simulink model "MotorPositionControl"  (R2020b)
settings: Solver=ode15s  StartTime=0.0  StopTime=0.2  RelTol=1e-3
undefined symbols (not defined in the file): b, J, kd, ke, ki, kp, kt, L, R
settings Model: DataDictionary=data_dict.sldd  Creator=Shree  LastModifiedBy=Shree

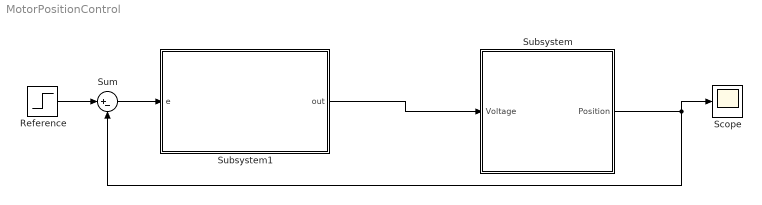
== system MotorPositionControl ==
  "Reference " : Step  Time=0.001  SampleTime=0
  Scope : Scope
  Subsystem : Subsystem
  Subsystem1 : Subsystem
  Sum : Sum  Inputs=|+-
  wires:
  Subsystem/1(Position) -> Scope/1, Sum/2
  Subsystem1/1(out) -> Subsystem/1(Voltage)
  "Reference "/1 -> Sum/1
  Sum/1 -> Subsystem1/1(e)

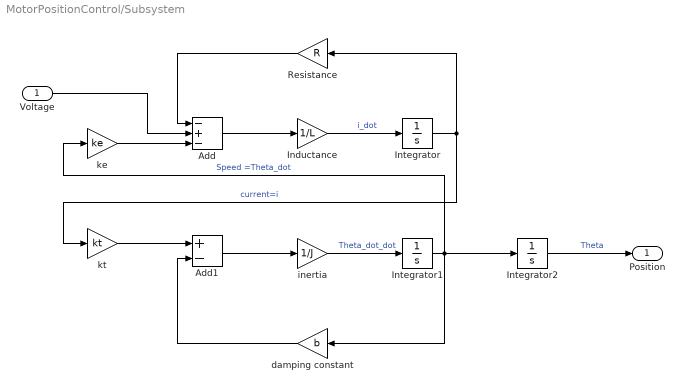
== system MotorPositionControl/Subsystem ==
  Voltage : Inport
  Add : Sum  Inputs=-+-
  Add1 : Sum  Inputs=+-
  Inductance : Gain  Gain=1/L
  Integrator : Integrator
  Integrator1 : Integrator
  Integrator2 : Integrator
  Resistance : Gain  Gain=R
  damping constant : Gain  Gain=b
  inertia : Gain  Gain=1/J
  ke : Gain  Gain=ke
  kt : Gain  Gain=kt
  Position : Outport
  wires:
  Inductance/1 -> Integrator/1  "i_dot"
  inertia/1 -> Integrator1/1  "Theta_dot_dot"
  Add1/1 -> inertia/1
  Integrator1/1 -> Integrator2/1, ke/1, damping constant/1  "Speed =Theta_dot"
  Integrator/1 -> Resistance/1, kt/1  "current=i"
  Resistance/1 -> Add/1
  kt/1 -> Add1/1
  damping constant/1 -> Add1/2
  Add/1 -> Inductance/1
  Integrator2/1 -> Position/1  "Theta"
  ke/1 -> Add/3
  Voltage/1 -> Add/2

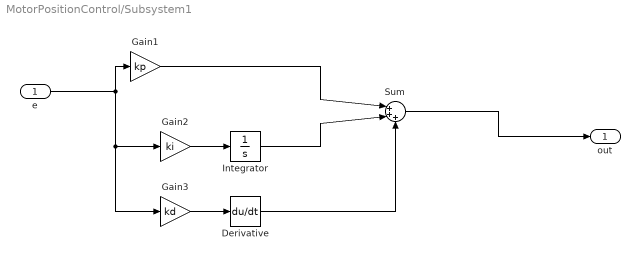
== system MotorPositionControl/Subsystem1 ==
  e : Inport
  Derivative : Derivative
  Gain1 : Gain  Gain=kp
  Gain2 : Gain  Gain=ki
  Gain3 : Gain  Gain=kd
  Integrator : Integrator
  Sum : Sum  Inputs=|+++
  out : Outport
  wires:
  Gain2/1 -> Integrator/1
  Gain3/1 -> Derivative/1
  Gain1/1 -> Sum/1
  Derivative/1 -> Sum/3
  Sum/1 -> out/1
  e/1 -> Gain3/1, Gain2/1, Gain1/1
  Integrator/1 -> Sum/2
